simulink model "Ch3"  (R2024b)
settings: Solver=VariableStepAuto  StartTime=0.0  StopTime=0.5  FixedStep=1E-4  RelTol=1e-5
libraries: spsSeriesRLCBranchLib x10, simulink x5, spsControlledCurrentSourceLib x3, spsVoltageMeasurementLib x3, spsDiodeLib x2, spspowerguiLib x2, spsIGBTLib x1, spsCurrentMeasurementLib x1, spsMosfetLib x1, sps_lib x1
settings Model: Creator=86195  LastModifiedBy=86195
settings DebuggingCC: AlgebraicLoopMsg=none

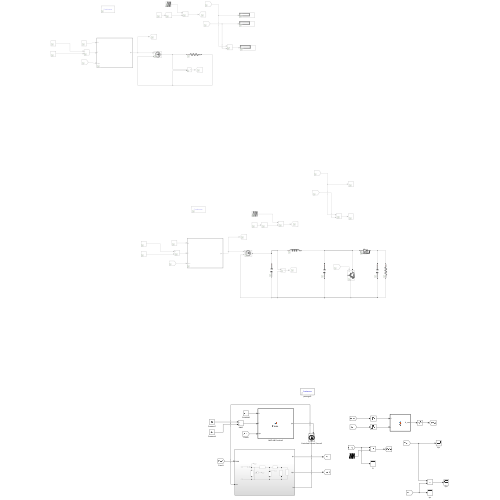
[thumbnail: Simulink's stored preview of the top-level diagram]
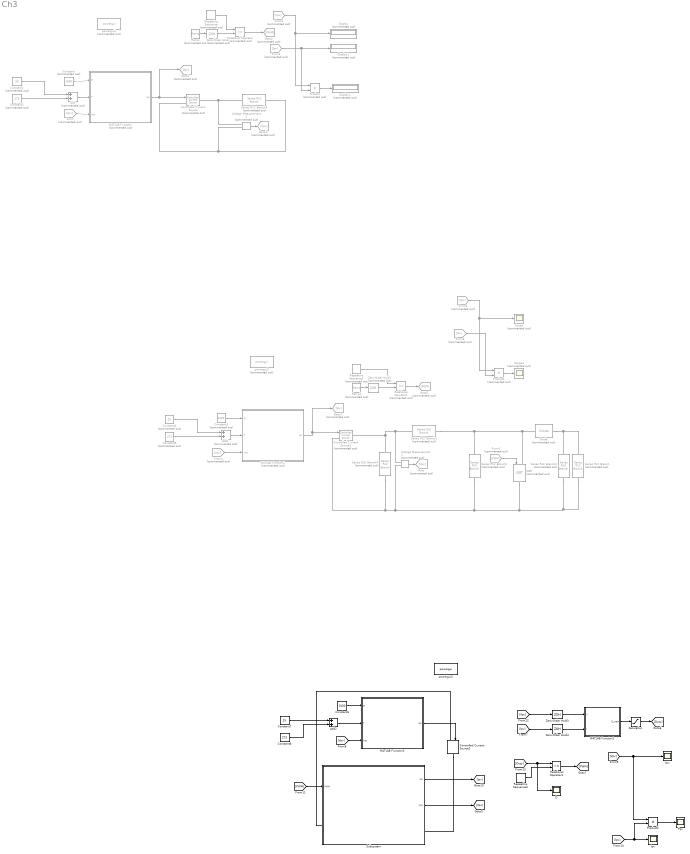
== system Ch3 ==
  Add : Sum  Commented=on
  Add1 : Sum  Commented=on
  Add2 : Sum
  Constant : Constant  Commented=on  Value=1000
  Constant1 : Constant  Commented=on  Value=50
  Constant2 : Constant  Commented=on  Value=273
  Constant3 : Constant  Commented=on  Value=1000
  Constant4 : Constant  Commented=on  Value=25
  Constant5 : Constant  Commented=on  Value=273
  Constant6 : Constant  Value=1000
  Constant7 : Constant  Value=25
  Constant8 : Constant  Value=273
  Controlled Current Source : spsControlledCurrentSourceLib/Controlled Current Source  Commented=on  Initialize=on  Source_Type=AC  Amplitude=0  Phase=0  Frequency=0  Measurements=None
  Controlled Current Source1 : spsControlledCurrentSourceLib/Controlled Current Source  Commented=on  Initialize=on  Source_Type=AC  Amplitude=0  Phase=0  Frequency=0  Measurements=None
  Controlled Current Source2 : spsControlledCurrentSourceLib/Controlled Current Source  Initialize=on  Source_Type=AC  Amplitude=0  Phase=0  Frequency=0  Measurements=None
  D : Scope
  Diode : spsDiodeLib/Diode  Commented=on  Ron=0.001  Lon=0  Vf=0.8  IC=0  UseSnubber=0  Rs=500  Cs=250e-9  Measurements=off
  Display : Display  Commented=on
  Display1 : Display  Commented=on
  Display2 : Display  Commented=on
  From{,2,4..5} (4 alike) : From  Commented=on  GotoTag=Vpv
  From1 : From  Commented=on  GotoTag=PWM
  From3 : From  Commented=on  GotoTag=Ipv
  From6 : From  Commented=on  GotoTag=Ipv
  Goto : Goto  Commented=on  GotoTag=Vpv
  Goto1 : Goto  Commented=on  GotoTag=Ipv
  Goto2 : Goto  Commented=on  GotoTag=PWM
  Goto3 : Goto  Commented=on  GotoTag=Vpv
  Goto4 : Goto  Commented=on  GotoTag=Ipv
  Goto5 : Goto  Commented=on  GotoTag=PWM
  IGBT : spsIGBTLib/IGBT  Commented=on  Ron=0.001  Lon=0  Vf=1  Tf=1e-6  Tt=2e-6  IC=0  Rs=1e5  Cs=inf  Measurements=off
  Ipv : Scope
  MATLAB Function : MATLAB Function  Commented=on  TreatAsAtomicUnit=on
  MATLAB Function1 : MATLAB Function  Commented=on  TreatAsAtomicUnit=on
  MATLAB Function2 : MATLAB Function  TreatAsAtomicUnit=on
  MATLAB Function3 : MATLAB Function  TreatAsAtomicUnit=on
  Ppv : Scope
  Product : Product  Commented=on
  Product1 : Product  Commented=on
  Product2 : Product
  Ramp : simulink/Sources/Ramp  Commented=on  slope=1  start=0  InitialOutput=0
  Ramp1 : simulink/Sources/Ramp  Commented=on  slope=-0.1  start=0  InitialOutput=0.5
  Relational Operator : RelationalOperator  Commented=on  Operator=<=  OutDataTypeStr=boolean  RndMeth=Simplest  InputSameDT=off
  Relational Operator1 : RelationalOperator  Commented=on  Operator=<=  OutDataTypeStr=boolean  RndMeth=Simplest  InputSameDT=off
  Relational Operator3 : RelationalOperator  OutDataTypeStr=boolean  RndMeth=Simplest  InputSameDT=off
  Repeating Sequence : simulink/Sources/Repeating Sequence  Commented=on  rep_seq_t=[0 1e-4]  rep_seq_y=[0 1]
  Repeating Sequence1 : simulink/Sources/Repeating Sequence  Commented=on  rep_seq_t=[0 1e-4]  rep_seq_y=[0 1]
  Repeating Sequence3 : simulink/Sources/Repeating Sequence  rep_seq_t=[0 1e-4]  rep_seq_y=[0 1]
  Saturation : Saturate
  Scope : Scope  Commented=on
  Scope1 : Scope  Commented=on
  Series RLC Branch : spsSeriesRLCBranchLib/Series RLC Branch  Commented=on  LConnTagsString=__new0  RConnTagsString=__new0  BranchType=R  Resistance=10  Inductance=1e-3  SetiL0=off  InitialCurrent=0  Capacitance=1e-6  Setx0=off  InitialVoltage=0  Measurements=None
  Series RLC Branch1 : spsSeriesRLCBranchLib/Series RLC Branch  Commented=on  LConnTagsString=__new0  RConnTagsString=__new0  BranchType=L  Resistance=1  Inductance=1e-3  SetiL0=off  InitialCurrent=0  Capacitance=1e-6  Setx0=off  InitialVoltage=0  Measurements=None
  Series RLC Branch2 : spsSeriesRLCBranchLib/Series RLC Branch  Commented=on  LConnTagsString=__new0  RConnTagsString=__new0  BranchType=C  Resistance=1  Inductance=1e-3  SetiL0=off  InitialCurrent=0  Capacitance=47*1e-6  Setx0=off  InitialVoltage=0  Measurements=None
  Series RLC Branch3 : spsSeriesRLCBranchLib/Series RLC Branch  Commented=on  LConnTagsString=__new0  RConnTagsString=__new0  BranchType=C  Resistance=1  Inductance=1e-3  SetiL0=off  InitialCurrent=0  Capacitance=47*1e-6  Setx0=off  InitialVoltage=0  Measurements=None
  Series RLC Branch4 : spsSeriesRLCBranchLib/Series RLC Branch  Commented=on  LConnTagsString=__new0  RConnTagsString=__new0  BranchType=C  Resistance=1  Inductance=1e-3  SetiL0=off  InitialCurrent=0  Capacitance=470*1e-6  Setx0=off  InitialVoltage=0  Measurements=None
  Series RLC Branch5 : spsSeriesRLCBranchLib/Series RLC Branch  Commented=on  LConnTagsString=__new0  RConnTagsString=__new0  BranchType=R  Resistance=10  Inductance=1e-3  SetiL0=off  InitialCurrent=0  Capacitance=1e-6  Setx0=off  InitialVoltage=0  Measurements=None
  Subsystem : Subsystem
  Voltage Measurement1 : spsVoltageMeasurementLib/Voltage Measurement  Commented=on  PhasorSimulation=off  OutputType=Complex  PSBequivalent=0
  Voltage Measurement2 : spsVoltageMeasurementLib/Voltage Measurement  Commented=on  PhasorSimulation=off  OutputType=Complex  PSBequivalent=0
  Vpv : Scope
  Zero-Order Hold : ZeroOrderHold  Commented=on  SampleTime=-1
  Zero-Order Hold1 : ZeroOrderHold  Commented=on  SampleTime=0.1
  Zero-Order Hold3 : ZeroOrderHold  SampleTime=0.01
  Zero-Order Hold4 : ZeroOrderHold  SampleTime=0.01
  powergui1 : spspowerguiLib/powergui  Priority=1  Commented=on  SimulationMode=Continuous  SampleTime=50e-6  frequency=60  Iterations=50  frequencyindice=0  Pbase=100e6  ErrMax=1e-4  UnitsV=kV  UnitsW=MW  buscounter=0  FunctionMessages=off  echomessages=off  EnableUseOfTLC=off  CurrentSourceSwitches=off  DisableSnubberDevices=off  DisableRonSwitches=off  DisableVfSwitches=off  DisplayEquations=off  AutomaticDiscreteSolvers=off  SolverType=Tustin/Backward Euler (TBE)  Interpol=off  ExternalGateDelay=off  methode=off  Ts=100  x0status=blocks  SPID=on  SwTol=0  HookPort=off  NonlinearTolerance=1e-4  nMaxIteration=100  ContinueOnMaxIteration=off  RestoreLinks=warning  ResistiveCurrentMeasurement=off  Frange=[0:2:500]  Ylog=off  Xlog=on  ShowGrid=off  save=off  variable=ZData  structure=0  ZoomFFT=off  StartTime=0.0  cycles=1  DisplayStyle=1  fundamental=60  FreqAxis=off  MaxFrequency=1000  frequencyindicesteady=1  RmsSteady=1  display=off
  powergui2 : spspowerguiLib/powergui  Priority=1  Commented=on  SimulationMode=Continuous  SampleTime=50e-6  frequency=60  Iterations=50  frequencyindice=0  Pbase=100e6  ErrMax=1e-4  UnitsV=kV  UnitsW=MW  buscounter=0  FunctionMessages=off  echomessages=off  EnableUseOfTLC=off  CurrentSourceSwitches=off  DisableSnubberDevices=off  DisableRonSwitches=off  DisableVfSwitches=off  DisplayEquations=off  AutomaticDiscreteSolvers=off  SolverType=Tustin/Backward Euler (TBE)  Interpol=off  ExternalGateDelay=off  methode=off  Ts=100  x0status=blocks  SPID=on  SwTol=0  HookPort=off  NonlinearTolerance=1e-4  nMaxIteration=100  ContinueOnMaxIteration=off  RestoreLinks=warning  ResistiveCurrentMeasurement=off  Frange=[0:2:500]  Ylog=off  Xlog=on  ShowGrid=off  save=off  variable=ZData  structure=0  ZoomFFT=off  StartTime=0.0  cycles=1  DisplayStyle=1  fundamental=60  FreqAxis=off  MaxFrequency=1000  frequencyindicesteady=1  RmsSteady=1  display=off
  powergui3 : sps_lib/powergui  Priority=1  SimulationMode=Continuous  SampleTime=50e-6  frequency=60  Iterations=50  frequencyindice=0  Pbase=100e6  ErrMax=1e-4  UnitsV=kV  UnitsW=MW  buscounter=0  FunctionMessages=off  echomessages=off  EnableUseOfTLC=off  CurrentSourceSwitches=off  DisableSnubberDevices=off  DisableRonSwitches=off  DisableVfSwitches=off  DisplayEquations=off  AutomaticDiscreteSolvers=off  SolverType=Tustin/Backward Euler (TBE)  Interpol=off  ExternalGateDelay=off  methode=off  Ts=100  x0status=blocks  SPID=on  SwTol=0  HookPort=off  NonlinearTolerance=1e-4  nMaxIteration=100  ContinueOnMaxIteration=off  RestoreLinks=warning  ResistiveCurrentMeasurement=off  Frange=[0:2:500]  Ylog=off  Xlog=on  ShowGrid=off  save=off  variable=ZData  structure=0  ZoomFFT=off  StartTime=0.0  cycles=1  DisplayStyle=1  fundamental=60  FreqAxis=off  MaxFrequency=1000  frequencyindicesteady=1  RmsSteady=1  display=off
  wires:
  Constant/1 -> MATLAB Function/1(G)
  Add/1 -> MATLAB Function/2(T)
  Constant1/1 -> Add/1
  Constant2/1 -> Add/2
  Repeating Sequence/1 -> Relational Operator/1
  MATLAB Function/1(Ipv) -> Goto1/1, Controlled Current Source/1
  From/1 -> MATLAB Function/3(Vpv)
  Ramp/1 -> Zero-Order Hold/1
  Zero-Order Hold/1 -> Relational Operator/2
  Relational Operator/1 -> Goto2/1
  From2/1 -> Product/1, Display/1
  From3/1 -> Product/2, Display1/1
  Product/1 -> Display2/1
  Voltage Measurement1/1 -> Goto3/1
  MATLAB Function1/1(Ipv) -> Goto4/1, Controlled Current Source1/1
  Constant3/1 -> MATLAB Function1/1(G)
  Constant5/1 -> Add1/2
  Zero-Order Hold1/1 -> Relational Operator1/2
  Relational Operator1/1 -> Goto5/1
  Ramp1/1 -> Zero-Order Hold1/1
  Add1/1 -> MATLAB Function1/2(T)
  Repeating Sequence1/1 -> Relational Operator1/1
  Product1/1 -> Scope1/1
  Constant4/1 -> Add1/1
  From5/1 -> Scope/1, Product1/1
  From4/1 -> MATLAB Function1/3(Vpv)
  From6/1 -> Product1/2
  Voltage Measurement2/1 -> Goto/1
  From1/1 -> IGBT/1
  MATLAB Function3/1(Ipv) -> Controlled Current Source2/1
  Constant7/1 -> Add2/1
  [Ipv] -> Product2/2, Ipv/1
  Add2/1 -> MATLAB Function3/2(T)
  Product2/1 -> Ppv/1
  Constant6/1 -> MATLAB Function3/1(G)
  Constant8/1 -> Add2/2
  [Vpv] -> Product2/1, Vpv/1
  [Vpv] -> MATLAB Function3/3(Vpv)
  Zero-Order Hold3/1 -> MATLAB Function2/1(V)
  Zero-Order Hold4/1 -> MATLAB Function2/2(I)
  MATLAB Function2/1(D_new) -> Saturation/1
  [Ipv] -> Zero-Order Hold4/1
  [Vpv] -> Zero-Order Hold3/1
  Saturation/1 -> [Duty]
  [Duty] -> D/1, Relational Operator3/1
  Repeating Sequence3/1 -> Relational Operator3/2
  Relational Operator3/1 -> [PWM]
  Subsystem/2(Vpv) -> [Vpv]
  Subsystem/1(Ipv) -> [Ipv]
  [PWM] -> Subsystem/1(PWM)
  connections:
  Series RLC Branch5/LConn1 -- Voltage Measurement1/LConn1 -- Controlled Current Source/RConn1
  Voltage Measurement1/LConn2 -- Controlled Current Source/LConn1 -- Series RLC Branch5/RConn1
  Voltage Measurement2/LConn1 -- Series RLC Branch4/LConn1 -- Controlled Current Source1/RConn1 -- Series RLC Branch1/LConn1
  Series RLC Branch3/RConn1 -- Series RLC Branch/RConn1 -- Series RLC Branch2/RConn1 -- Series RLC Branch4/RConn1 -- Controlled Current Source1/LConn1 -- Voltage Measurement2/LConn2 -- IGBT/RConn1
  IGBT/LConn1 -- Diode/LConn1 -- Series RLC Branch2/LConn1 -- Series RLC Branch1/RConn1
  Diode/RConn1 -- Series RLC Branch/LConn1 -- Series RLC Branch3/LConn1
  Controlled Current Source2/LConn1 -- Subsystem/LConn1
  Controlled Current Source2/RConn1 -- Subsystem/RConn1

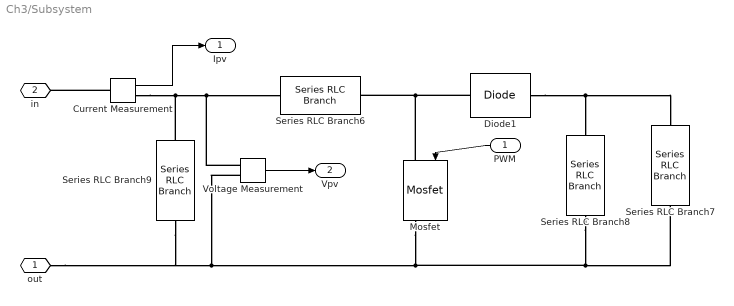
== system Ch3/Subsystem ==
  PWM : Inport
  Current Measurement : spsCurrentMeasurementLib/Current Measurement  PhasorSimulation=off  OutputType=Complex  PSBequivalent=0
  Diode1 : spsDiodeLib/Diode  Ron=0.001  Lon=0  Vf=0.8  IC=0  UseSnubber=0  Rs=500  Cs=250e-9  Measurements=off
  Mosfet : spsMosfetLib/Mosfet  Ron=0.1  Lon=0  Rd=0.01  Vfd=0  IC=0  Rs=1e5  Cs=inf  Measurements=on
  Series RLC Branch6 : spsSeriesRLCBranchLib/Series RLC Branch  LConnTagsString=__new0  RConnTagsString=__new0  BranchType=L  Resistance=1  Inductance=1e-3  SetiL0=off  InitialCurrent=0  Capacitance=1e-6  Setx0=off  InitialVoltage=0  Measurements=None
  Series RLC Branch7 : spsSeriesRLCBranchLib/Series RLC Branch  LConnTagsString=__new0  RConnTagsString=__new0  BranchType=R  Resistance=10  Inductance=1e-3  SetiL0=off  InitialCurrent=0  Capacitance=1e-6  Setx0=off  InitialVoltage=0  Measurements=None
  Series RLC Branch8 : spsSeriesRLCBranchLib/Series RLC Branch  LConnTagsString=__new0  RConnTagsString=__new0  BranchType=C  Resistance=1  Inductance=1e-3  SetiL0=off  InitialCurrent=0  Capacitance=47*1e-6  Setx0=off  InitialVoltage=0  Measurements=None
  Series RLC Branch9 : spsSeriesRLCBranchLib/Series RLC Branch  LConnTagsString=__new0  RConnTagsString=__new0  BranchType=C  Resistance=1  Inductance=1e-3  SetiL0=off  InitialCurrent=0  Capacitance=47*1e-6  Setx0=off  InitialVoltage=0  Measurements=None
  Voltage Measurement : spsVoltageMeasurementLib/Voltage Measurement  PhasorSimulation=off  OutputType=Complex  PSBequivalent=0
  out : PMIOPort  Side=Left
  in : PMIOPort  Port=2  Side=Right
  Ipv : Outport
  Vpv : Outport  Port=2
  wires:
  PWM/1 -> Mosfet/1
  Voltage Measurement/1 -> Vpv/1
  Current Measurement/1 -> Ipv/1
  connections:
  Series RLC Branch9/LConn1 -- Current Measurement/RConn1 -- Series RLC Branch6/LConn1 -- Voltage Measurement/LConn1
  Series RLC Branch8/RConn1 -- Series RLC Branch7/RConn1 -- out/RConn1 -- Series RLC Branch9/RConn1 -- Voltage Measurement/LConn2 -- Mosfet/RConn1
  Diode1/RConn1 -- Series RLC Branch7/LConn1 -- Series RLC Branch8/LConn1
  Diode1/LConn1 -- Mosfet/LConn1 -- Series RLC Branch6/RConn1
  Current Measurement/LConn1 -- in/RConn1

== matlab function Ch3/MATLAB Function ==
  data: G input; Ipv output; T input; Vpv input
function Ipv = EN50530(G,T,Vpv)
%% 光伏电池EN50530模型搭建
%% 光伏电池制造商所提供的参数
Isc0 = 3.8;  %标准工况下的短路电流
Voc0 = 21.1;  %标准工况下的开路电压
%% EN50530参数
G0 = 1000;  %光照强度
T0 = 25+273;  %光伏电池温度
a = 0.0004;
b = -0.004;
FFV = 0.8;
FFI = 0.9;
CG = 2.514e-3;
CV = 8.593e-2;
CR = 1.088e-4;

%% EN50530 公式计算
CAQ = (FFV-1)/log(1-FFI);
Isc = (G/G0)*Isc0*(1+a*(T-T0));
Voc = Voc0*(1+b*(T-T0))*(log(G/CG+1)*CV - CR*G);
I0 = (G/G0)*Isc0*(1-FFI)^(1/(1-FFV));
Ipv = Isc - I0*(exp(Vpv/(Voc*CAQ))-1); %计算光伏组件的电流

== matlab function Ch3/MATLAB Function2 ==
  data: V input; D_new output; I input
function D_new = PO(V, I)
%% 定义静态变量
persistent V_old P_old D_old;
%% 初始化静态变量
if(isempty(V_old))
    V_old = 0;
    P_old = 0;
    D_old = 0.4;
end
%% 更新电压、功率数据
P = V*I;
dP = P-P_old;
dV = V-V_old;
%% 步长方向判断
if (dP>0)
    if (dV>0)
        step = -0.02;
    else
        step = 0.02;
    end
else
    if (dV>0)
        step = 0.02;
    else
        step = -0.02;
    end
end
%% 更新占空比
D_new = D_old + step;
%% 将当前电压、功率、占空比保存到下一次
D_old = D_new;
V_old = V;
P_old = P;

== matlab function Ch3/MATLAB Function3 ==
  data: G input; Ipv output; T input; Vpv input
function Ipv = EN50530(G,T,Vpv)
%% 光伏电池EN50530模型搭建
%% 光伏电池制造商所提供的参数
Isc0 = 3.8;  %标准工况下的短路电流
Voc0 = 21.1;  %标准工况下的开路电压
%% EN50530参数
G0 = 1000;  %光照强度
T0 = 25+273;  %光伏电池温度
a = 0.0004;
b = -0.004;
FFV = 0.8;
FFI = 0.9;
CG = 2.514e-3;
CV = 8.593e-2;
CR = 1.088e-4;

%% EN50530 公式计算
CAQ = (FFV-1)/log(1-FFI);
Isc = (G/G0)*Isc0*(1+a*(T-T0));
Voc = Voc0*(1+b*(T-T0))*(log(G/CG+1)*CV - CR*G);
I0 = (G/G0)*Isc0*(1-FFI)^(1/(1-FFV));
Ipv = Isc - I0*(exp(Vpv/(Voc*CAQ))-1); %计算光伏组件的电流

== matlab function Ch3/MATLAB Function1 ==
  data: G input; Ipv output; T input; Vpv input
function Ipv = EN50530(G,T,Vpv)
%% 光伏电池EN50530模型搭建
%% 光伏电池制造商所提供的参数
Isc0 = 3.8;  %标准工况下的短路电流
Voc0 = 21.1;  %标准工况下的开路电压
%% EN50530参数
G0 = 1000;  %光照强度
T0 = 25+273;  %光伏电池温度
a = 0.0004;
b = -0.004;
FFV = 0.8;
FFI = 0.9;
CG = 2.514e-3;
CV = 8.593e-2;
CR = 1.088e-4;

%% EN50530 公式计算
CAQ = (FFV-1)/log(1-FFI);
Isc = (G/G0)*Isc0*(1+a*(T-T0));
Voc = Voc0*(1+b*(T-T0))*(log(G/CG+1)*CV - CR*G);
I0 = (G/G0)*Isc0*(1-FFI)^(1/(1-FFV));
Ipv = Isc - I0*(exp(Vpv/(Voc*CAQ))-1); %计算光伏组件的电流
